simulink model "FinalRobot"  (R2021b)
settings: Solver=ode23t  StartTime=0.0  StopTime=120  MaxStep=3e-3  RelTol=1e-3
undefined symbols (not defined in the file): Amor1, Amor2, Amor3, Amor4, Amor5, B_Verin1, B_Verin2, B_Verin3, B_Verin4, B_Verin5, H_Verin1, H_Verin2, H_Verin3, H_Verin4, H_Verin5, k, K, Middle_Sensing, Sensing_1, Sensing_2, Wall_1, Wall_10, Wall_11, Wall_2, Wall_3, Wall_4, Wall_5, Wall_6, Wall_7, Wall_8, Wall_9, X, Y, Z
libraries: sm_lib x237, nesl_utility x60
(part 3 of 8)

== system FinalRobot/Snake/Verin2 ==
  Tor32 : Inport
  Torq31 : Inport  Port=2
  Camera : sm_lib/Body Elements/Spherical Solid  GraphicAmbientColor=[0.15 0.15 0.15 1.0]  BasedOnType=Density  CenterOfMass=[0 0 0]  CenterOfMassUnits=m  GraphicDiffuseColor=[0.9411765 0.9411765 0.9411765]  Density=10  DensityUnits=kg/m^3  DoExposeReferenceFrame=on  GraphicEmissiveColor=[0.0 0.0 0.0 1.0]  ExportEntireGeometry=off  SerializedExposedGeometries=<ExposedGeometries/>  SerializedFrames=<Frames/>  MarkerShape=Sphere  MarkerSize=10  GraphicType=FromGeometry  InertiaType=CalculateFromGeometry  Mass=1  MassUnits=kg  MomentsOfInertia=[1 1 1]  MomentsOfInertiaUnits=kg*m^2  GraphicOpacity=0  ProductsOfInertia=[0 0 0]  ProductsOfInertiaUnits=kg*m^2  GraphicShininess=75  GraphicSpecularColor=[0.5 0.5 0.5 1.0]  SphereRadius=0.1  SphereRadiusUnits=cm  GraphicVisPropType=SimpleVisualProperties
  Revolute Joint1 : sm_lib/Joints/Revolute Joint  JointMode=Normal  SenseConstraintForce=off  SenseConstraintForceX=off  SenseConstraintForceY=off  SenseConstraintForceZ=off  SenseConstraintTorque=off  SenseConstraintTorqueX=off  SenseConstraintTorqueY=off  SenseConstraintTorqueZ=off  SenseTotalForce=off  SenseTotalForceX=off  SenseTotalForceY=off  SenseTotalForceZ=off  SenseTotalTorque=off  SenseTotalTorqueX=off  SenseTotalTorqueY=off  SenseTotalTorqueZ=off  CompositeWrenchDir=FollowerOnBase  CompositeWrenchFrame=BaseFrame  EquilibriumPosition=0  EquilibriumPositionUnits=deg  SpringStiffness=Stiffness_Spine  SpringStiffnessUnits=N*m/deg  DampingCoefficient=Damping_Spine  DampingCoefficientUnits=N*m/(deg/s)  TorqueActuationMode=NoTorque  MotionActuationMode=ComputedMotion  SensePosition=off  SenseVelocity=off  SenseAcceleration=off  SenseTorqueForce=off  SenseLowerLimitTorqueForce=off  SenseUpperLimitTorqueForce=off  LowerLimitSpecify=off  LowerLimitBound=-90  LowerLimitBoundUnits=deg  LowerLimitStiffness=1e4  LowerLimitStiffnessUnits=N*m/deg  LowerLimitDamping=10  LowerLimitDampingUnits=N*m/(deg/s)  LowerLimitTransitionRegionWidth=0.1  LowerLimitTransitionRegionWidthUnits=deg  UpperLimitSpecify=off  UpperLimitBound=90  UpperLimitBoundUnits=deg  UpperLimitStiffness=1e4  UpperLimitStiffnessUnits=N*m/deg  UpperLimitDamping=10  UpperLimitDampingUnits=N*m/(deg/s)  UpperLimitTransitionRegionWidth=0.1  UpperLimitTransitionRegionWidthUnits=deg  PositionTargetSpecify=off  PositionTargetPriority=High  PositionTargetValue=0  PositionTargetValueUnits=deg  VelocityTargetSpecify=off  VelocityTargetPriority=High  VelocityTargetValue=0  VelocityTargetValueUnits=deg/s
  Rigid Transform4 : sm_lib/Frames and Transforms/Rigid Transform  TranslationMethod=Cartesian  TranslationStandardOffset=-10  TranslationLengthUnit=m  TranslationStandardAxis=+Z  TranslationCartesianOffset=[0 -0.1 0.1]  TranslationROffset=0  TranslationROffsetUnits=m  TranslationZOffset=0  TranslationZOffsetUnits=m  TranslationThetaOffset=0  TranslationThetaOffsetUnits=deg  RotationMethod=StandardAxis  RotationAngleUnits=deg  RotationStandardAxis=+Z  RotationAngle=-10  RotationArbitraryAxis=[0 0 1]  FollAlignAxisA=+X  BaseAlignAxisA=+Y  FollAlignAxisB=+Y  BaseAlignAxisB=+Z  RotationSequenceAxes=FollowerAxes  RotationSequence=XYX  RotationSequenceAngles=[-45 45 0]  RotationSequenceAnglesUnits=deg  RotationMatrix=[1 0 0; 0 1 0; 0 0 1]
  Subsystem1 : Subsystem
      mask Display: image('C:\Users\MINGO Monique\Pictures\MatLab images\MatLab_img3.PNG'); % Use "Edit Image" on toolstrip to change.
  Subsystem3 : Subsystem
      settings: PortSchema="{\"entries\":[{\"content\":{\"sides\":[{\"content\":{\"connectorIds\":[\"LConn1\"]},\"type\":\"ConnectorPlacement.EquallySpacedRectSide\",\"uuid\":\"fb7ca892-623b-4289-934f-aee105276814\"},{\"content\":{\"connectorIds\":[\"RConn1\"],\"side\":\"RIGHT\"},\"type\":\"ConnectorPlacement.EquallySpacedRectSide\",\"uuid\":\"0daf8b48-229f-46bb-9482-184447c743c5\"},{\"content\":{\"connectorIds\":[\"In1\",\"In2\",\"Out1\",\"Out2\"],\"side\":\"TOP\"},\"type\":\"ConnectorPlacement.EquallySpacedRectSide\",\"uuid\":\"c258a386-6c23-4ebb-b6ca-e534711f920f\"},{\"content\":{\"connectorIds\":[\"RConn2\",\"RConn3\",\"RConn4\",\"RConn5\"],\"side\":\"BOTTOM\"},\"type\":\"ConnectorPlacement.EquallySpacedRectSide\",\"uuid\":\"3e83ec0e-900d-4924-8cc6-19cde9453293\"}]},\"type\":\"ConnectorPlacement.EquallySpacedConnector\",\"uuid\":\"dfcdae3d-d414-45a1-b62e-1dc7d14d079d\"}],\"packageUris\":[\"http://schema.mathworks.com/mf0/Connector/R2020b\"],\"version\":\"1.0\"}"
      mask Display: image('$imagefile'); % Use "Edit Image" on toolstrip to change.
  Subsystem5 : Subsystem
      mask Display: image('C:\Users\MINGO Monique\Pictures\MatLab images\MatLab_img2.PNG'); % Use "Edit Image" on toolstrip to change.
  Conn1 : PMIOPort  Side=Left
  Conn7 : PMIOPort  Port=2  Side=Right
  Conn3 : PMIOPort  Port=3  Side=Right
  Amor : PMIOPort  Port=4  Side=Right
  Conn4 : PMIOPort  Port=5  Side=Right
  Conn2 : PMIOPort  Port=6  Side=Right
  Ref2 : PMIOPort  Port=7  Side=Right
  Ref3 : PMIOPort  Port=8  Side=Right
  azm3 : Outport
  wz3 : Outport  Port=2
  wires:
  Torq31/1 -> Subsystem3/2(input1)
  Tor32/1 -> Subsystem3/1(input0)
  Subsystem3/1(azm3) -> azm3/1
  Subsystem3/2(wz3) -> wz3/1
  connections:
  Subsystem3/RConn4 -- Conn2/RConn1
  Subsystem3/RConn3 -- Conn4/RConn1
  Subsystem3/RConn2 -- Amor/RConn1
  Conn7/RConn1 -- Subsystem1/LConn1 -- Subsystem3/RConn1
  Subsystem3/LConn1 -- Conn1/RConn1
  Conn3/RConn1 -- Rigid Transform4/LConn1 -- Subsystem5/RConn1
  Ref3/RConn1 -- Subsystem1/RConn1 -- Revolute Joint1/RConn1
  Revolute Joint1/LConn1 -- Subsystem5/LConn1
  Ref2/RConn1 -- Subsystem3/RConn5
  Camera/RConn1 -- Rigid Transform4/RConn1

== system FinalRobot/Snake/Verin3 ==
  Tor42 : Inport
  Torq41 : Inport  Port=2
  Revolute Joint1 : sm_lib/Joints/Revolute Joint  JointMode=Normal  SenseConstraintForce=off  SenseConstraintForceX=off  SenseConstraintForceY=off  SenseConstraintForceZ=off  SenseConstraintTorque=off  SenseConstraintTorqueX=off  SenseConstraintTorqueY=off  SenseConstraintTorqueZ=off  SenseTotalForce=off  SenseTotalForceX=off  SenseTotalForceY=off  SenseTotalForceZ=off  SenseTotalTorque=off  SenseTotalTorqueX=off  SenseTotalTorqueY=off  SenseTotalTorqueZ=off  CompositeWrenchDir=FollowerOnBase  CompositeWrenchFrame=BaseFrame  EquilibriumPosition=0  EquilibriumPositionUnits=deg  SpringStiffness=Stiffness_Spine  SpringStiffnessUnits=N*m/deg  DampingCoefficient=Damping_Spine  DampingCoefficientUnits=N*m/(deg/s)  TorqueActuationMode=NoTorque  MotionActuationMode=ComputedMotion  SensePosition=off  SenseVelocity=off  SenseAcceleration=off  SenseTorqueForce=off  SenseLowerLimitTorqueForce=off  SenseUpperLimitTorqueForce=off  LowerLimitSpecify=off  LowerLimitBound=-90  LowerLimitBoundUnits=deg  LowerLimitStiffness=1e4  LowerLimitStiffnessUnits=N*m/deg  LowerLimitDamping=10  LowerLimitDampingUnits=N*m/(deg/s)  LowerLimitTransitionRegionWidth=0.1  LowerLimitTransitionRegionWidthUnits=deg  UpperLimitSpecify=off  UpperLimitBound=90  UpperLimitBoundUnits=deg  UpperLimitStiffness=1e4  UpperLimitStiffnessUnits=N*m/deg  UpperLimitDamping=10  UpperLimitDampingUnits=N*m/(deg/s)  UpperLimitTransitionRegionWidth=0.1  UpperLimitTransitionRegionWidthUnits=deg  PositionTargetSpecify=off  PositionTargetPriority=High  PositionTargetValue=0  PositionTargetValueUnits=deg  VelocityTargetSpecify=off  VelocityTargetPriority=High  VelocityTargetValue=0  VelocityTargetValueUnits=deg/s
  Subsystem1 : Subsystem
      mask Display: image('C:\Users\MINGO Monique\Pictures\MatLab images\MatLab_img3.PNG'); % Use "Edit Image" on toolstrip to change.
  Subsystem3 : Subsystem
      settings: PortSchema="{\"entries\":[{\"content\":{\"sides\":[{\"content\":{\"connectorIds\":[\"LConn1\"]},\"type\":\"ConnectorPlacement.EquallySpacedRectSide\",\"uuid\":\"fb7ca892-623b-4289-934f-aee105276814\"},{\"content\":{\"connectorIds\":[\"RConn1\"],\"side\":\"RIGHT\"},\"type\":\"ConnectorPlacement.EquallySpacedRectSide\",\"uuid\":\"0daf8b48-229f-46bb-9482-184447c743c5\"},{\"content\":{\"connectorIds\":[\"In1\",\"In2\",\"Out1\",\"Out2\"],\"side\":\"TOP\"},\"type\":\"ConnectorPlacement.EquallySpacedRectSide\",\"uuid\":\"c258a386-6c23-4ebb-b6ca-e534711f920f\"},{\"content\":{\"connectorIds\":[\"RConn2\",\"RConn3\",\"RConn4\",\"RConn5\"],\"side\":\"BOTTOM\"},\"type\":\"ConnectorPlacement.EquallySpacedRectSide\",\"uuid\":\"3e83ec0e-900d-4924-8cc6-19cde9453293\"}]},\"type\":\"ConnectorPlacement.EquallySpacedConnector\",\"uuid\":\"dfcdae3d-d414-45a1-b62e-1dc7d14d079d\"}],\"packageUris\":[\"http://schema.mathworks.com/mf0/Connector/R2020b\"],\"version\":\"1.0\"}"
      mask Display: image('$imagefile'); % Use "Edit Image" on toolstrip to change.
  Subsystem5 : Subsystem
      mask Display: image('C:\Users\MINGO Monique\Pictures\MatLab images\MatLab_img2.PNG'); % Use "Edit Image" on toolstrip to change.
  Conn1 : PMIOPort  Side=Left
  Conn3 : PMIOPort  Port=2  Side=Right
  Amor : PMIOPort  Port=3  Side=Right
  Conn4 : PMIOPort  Port=4  Side=Right
  Conn2 : PMIOPort  Port=5  Side=Right
  Ref3 : PMIOPort  Port=6  Side=Right
  Ref4 : PMIOPort  Port=7  Side=Right
  azm4 : Outport
  wz4 : Outport  Port=2
  wires:
  Tor42/1 -> Subsystem3/1(input0)
  Torq41/1 -> Subsystem3/2(input1)
  Subsystem3/1(azm4) -> azm4/1
  Subsystem3/2(wz4) -> wz4/1
  connections:
  Subsystem3/LConn1 -- Conn1/RConn1
  Subsystem3/RConn2 -- Amor/RConn1
  Subsystem3/RConn3 -- Conn4/RConn1
  Subsystem3/RConn4 -- Conn2/RConn1
  Ref4/RConn1 -- Subsystem1/RConn1 -- Revolute Joint1/RConn1
  Revolute Joint1/LConn1 -- Subsystem5/LConn1
  Subsystem1/LConn1 -- Subsystem3/RConn1
  Ref3/RConn1 -- Subsystem3/RConn5
  Conn3/RConn1 -- Subsystem5/RConn1

== system FinalRobot/Snake/Verin4 ==
  Tor52 : Inport
  Torq51 : Inport  Port=2
  Subsystem1 : Subsystem
      settings: PortSchema="{\"entries\":[{\"content\":{\"sides\":[{\"content\":{\"connectorIds\":[\"LConn1\"]},\"type\":\"ConnectorPlacement.EquallySpacedRectSide\",\"uuid\":\"fb7ca892-623b-4289-934f-aee105276814\"},{\"content\":{\"connectorIds\":[\"RConn1\"],\"side\":\"RIGHT\"},\"type\":\"ConnectorPlacement.EquallySpacedRectSide\",\"uuid\":\"0daf8b48-229f-46bb-9482-184447c743c5\"},{\"content\":{\"connectorIds\":[\"In1\",\"In2\",\"Out1\",\"Out2\"],\"side\":\"TOP\"},\"type\":\"ConnectorPlacement.EquallySpacedRectSide\",\"uuid\":\"c258a386-6c23-4ebb-b6ca-e534711f920f\"},{\"content\":{\"connectorIds\":[\"RConn2\",\"RConn3\",\"RConn4\",\"RConn5\"],\"side\":\"BOTTOM\"},\"type\":\"ConnectorPlacement.EquallySpacedRectSide\",\"uuid\":\"3e83ec0e-900d-4924-8cc6-19cde9453293\"}]},\"type\":\"ConnectorPlacement.EquallySpacedConnector\",\"uuid\":\"dfcdae3d-d414-45a1-b62e-1dc7d14d079d\"}],\"packageUris\":[\"http://schema.mathworks.com/mf0/Connector/R2020b\"],\"version\":\"1.0\"}"
      mask Display: image('$imagefile'); % Use "Edit Image" on toolstrip to change.
  Conn1 : PMIOPort  Side=Left
  Amor : PMIOPort  Port=2  Side=Right
  Conn4 : PMIOPort  Port=3  Side=Right
  Conn2 : PMIOPort  Port=4  Side=Right
  Ref4 : PMIOPort  Port=5  Side=Right
  azm5 : Outport
  wz5 : Outport  Port=2
  wires:
  Torq51/1 -> Subsystem1/2(input1)
  Tor52/1 -> Subsystem1/1(input0)
  Subsystem1/1(azm5) -> azm5/1
  Subsystem1/2(wz5) -> wz5/1
  connections:
  Subsystem1/RConn4 -- Conn2/RConn1
  Subsystem1/RConn3 -- Conn4/RConn1
  Subsystem1/RConn2 -- Amor/RConn1
  Subsystem1/LConn1 -- Conn1/RConn1
  Ref4/RConn1 -- Subsystem1/RConn5

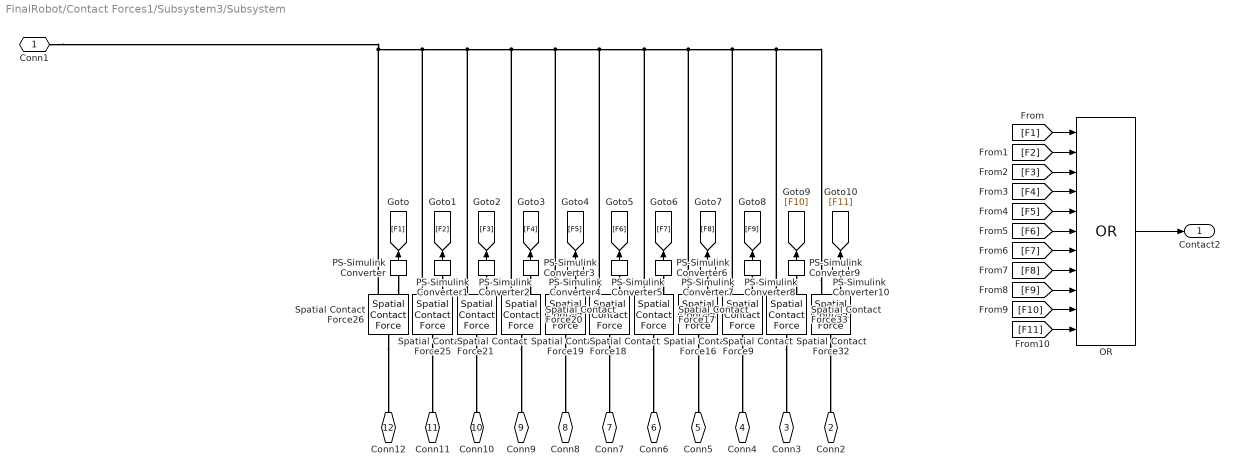
== system FinalRobot/Contact Forces1/Subsystem3/Subsystem ==
  OR : Logic  Operator=OR  Inputs=11  IconShape=distinctive  AllPortsSameDT=off  OutDataTypeStr=boolean
  PS-Simulink Converter{,1..10} (11 alike) : nesl_utility/PS-Simulink Converter  PhysicalDomain=network_engine_domain  SubClassName=ps_output  LeftPortType=input  RightPortType=output  PseudoPeriodic=off  Frequencies=[]  Unit=inherit  AffineConversion=off
      settings: SourceProductBaseCode=PW,SS
  Spatial Contact Force{9,16..21,25..26,32..33} (11 alike) : sm_lib/Forces and Torques/Spatial Contact Force  CoefficientOfDynamicFriction=0.3  CoefficientOfStaticFriction=0.5  SenseContactBaseRotation=off  SenseContactBaseTranslation=off  NormalDamping=1e3  NormalDampingUnits=N/(m/s)  SenseContactFollowerRotation=off  SenseContactFollowerTranslation=off  SenseContactSignal=off  NormalStiffness=1e6  NormalStiffnessUnits=N/m  FrictionalCriticalVelocity=1e-3  FrictionalCriticalVelocityUnits=m/s  ZeroCrossDetectContactStartAndEnd=off  FrictionType=SmoothStickSlip  SenseFrictionalForceMagnitude=off  SenseNormalForceMagnitude=on  NormalForceType=SmoothSpringDamper  SenseNormalVelocity=off  SenseSeparationDistance=off  SenseTangentialVelocity=off  SenseTangentialVelocityMagnitude=off  NormalTransitionRegionWidth=1e-4  NormalTransitionRegionWidthUnits=m
  Conn1 : PMIOPort  Side=Left
  Conn2 : PMIOPort  Port=2  Side=Right
  Conn3 : PMIOPort  Port=3  Side=Right
  Conn4 : PMIOPort  Port=4  Side=Right
  Conn5 : PMIOPort  Port=5  Side=Right
  Conn6 : PMIOPort  Port=6  Side=Right
  Conn7 : PMIOPort  Port=7  Side=Right
  Conn8 : PMIOPort  Port=8  Side=Right
  Conn9 : PMIOPort  Port=9  Side=Right
  Conn10 : PMIOPort  Port=10  Side=Right
  Conn11 : PMIOPort  Port=11  Side=Right
  Conn12 : PMIOPort  Port=12  Side=Right
  Contact2 : Outport
  wires:
  PS-Simulink Converter8/1 -> [F9]
  PS-Simulink Converter9/1 -> [F10]
  [F11] -> OR/11
  [F7] -> OR/7
  [F6] -> OR/6
  PS-Simulink Converter1/1 -> [F2]
  OR/1 -> Contact2/1
  [F2] -> OR/2
  PS-Simulink Converter4/1 -> [F5]
  [F4] -> OR/4
  PS-Simulink Converter7/1 -> [F8]
  [F10] -> OR/10
  [F3] -> OR/3
  [F1] -> OR/1
  PS-Simulink Converter2/1 -> [F3]
  PS-Simulink Converter3/1 -> [F4]
  [F8] -> OR/8
  PS-Simulink Converter/1 -> [F1]
  PS-Simulink Converter10/1 -> [F11]
  [F9] -> OR/9
  PS-Simulink Converter6/1 -> [F7]
  PS-Simulink Converter5/1 -> [F6]
  [F5] -> OR/5
  connections:
  Spatial Contact Force33/LConn1 -- Conn3/RConn1
  PS-Simulink Converter6/LConn1 -- Spatial Contact Force17/RConn2
  PS-Simulink Converter4/LConn1 -- Spatial Contact Force19/RConn2
  Spatial Contact Force9/RConn2 -- PS-Simulink Converter8/LConn1
  PS-Simulink Converter9/LConn1 -- Spatial Contact Force33/RConn2
  Spatial Contact Force18/LConn1 -- Conn7/RConn1
  PS-Simulink Converter1/LConn1 -- Spatial Contact Force25/RConn2
  Spatial Contact Force32/RConn1 -- Conn1/RConn1 -- Spatial Contact Force26/RConn1 -- Spatial Contact Force25/RConn1 -- Spatial Contact Force21/RConn1 -- Spatial Contact Force20/RConn1 -- Spatial Contact Force19/RConn1 -- Spatial Contact Force18/RConn1 -- Spatial Contact Force17/RConn1 -- Spatial Contact Force16/RConn1 -- Spatial Contact Force9/RConn1 -- Spatial Contact Force33/RConn1
  PS-Simulink Converter7/LConn1 -- Spatial Contact Force16/RConn2
  Spatial Contact Force16/LConn1 -- Conn5/RConn1
  PS-Simulink Converter5/LConn1 -- Spatial Contact Force18/RConn2
  Spatial Contact Force20/LConn1 -- Conn9/RConn1
  PS-Simulink Converter2/LConn1 -- Spatial Contact Force21/RConn2
  PS-Simulink Converter/LConn1 -- Spatial Contact Force26/RConn2
  Spatial Contact Force21/LConn1 -- Conn10/RConn1
  Spatial Contact Force17/LConn1 -- Conn6/RConn1
  Spatial Contact Force19/LConn1 -- Conn8/RConn1
  PS-Simulink Converter10/LConn1 -- Spatial Contact Force32/RConn2
  PS-Simulink Converter3/LConn1 -- Spatial Contact Force20/RConn2
  Spatial Contact Force25/LConn1 -- Conn11/RConn1
  Spatial Contact Force26/LConn1 -- Conn12/RConn1
  Spatial Contact Force32/LConn1 -- Conn2/RConn1
  Spatial Contact Force9/LConn1 -- Conn4/RConn1

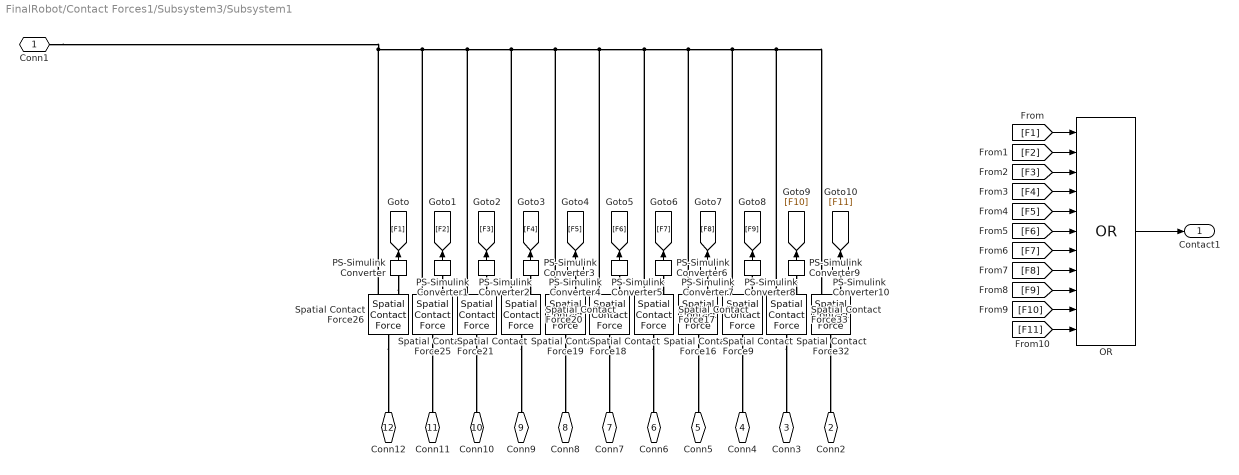
== system FinalRobot/Contact Forces1/Subsystem3/Subsystem1 ==
  OR : Logic  Operator=OR  Inputs=11  IconShape=distinctive  AllPortsSameDT=off  OutDataTypeStr=boolean
  PS-Simulink Converter{,1..10} (11 alike) : nesl_utility/PS-Simulink Converter  PhysicalDomain=network_engine_domain  SubClassName=ps_output  LeftPortType=input  RightPortType=output  PseudoPeriodic=off  Frequencies=[]  Unit=inherit  AffineConversion=off
      settings: SourceProductBaseCode=PW,SS
  Spatial Contact Force{9,16..21,25..26,32..33} (11 alike) : sm_lib/Forces and Torques/Spatial Contact Force  CoefficientOfDynamicFriction=0.3  CoefficientOfStaticFriction=0.5  SenseContactBaseRotation=off  SenseContactBaseTranslation=off  NormalDamping=1e3  NormalDampingUnits=N/(m/s)  SenseContactFollowerRotation=off  SenseContactFollowerTranslation=off  SenseContactSignal=off  NormalStiffness=1e6  NormalStiffnessUnits=N/m  FrictionalCriticalVelocity=1e-3  FrictionalCriticalVelocityUnits=m/s  ZeroCrossDetectContactStartAndEnd=off  FrictionType=SmoothStickSlip  SenseFrictionalForceMagnitude=off  SenseNormalForceMagnitude=on  NormalForceType=SmoothSpringDamper  SenseNormalVelocity=off  SenseSeparationDistance=off  SenseTangentialVelocity=off  SenseTangentialVelocityMagnitude=off  NormalTransitionRegionWidth=1e-4  NormalTransitionRegionWidthUnits=m
  Conn1 : PMIOPort  Side=Left
  Conn2 : PMIOPort  Port=2  Side=Right
  Conn3 : PMIOPort  Port=3  Side=Right
  Conn4 : PMIOPort  Port=4  Side=Right
  Conn5 : PMIOPort  Port=5  Side=Right
  Conn6 : PMIOPort  Port=6  Side=Right
  Conn7 : PMIOPort  Port=7  Side=Right
  Conn8 : PMIOPort  Port=8  Side=Right
  Conn9 : PMIOPort  Port=9  Side=Right
  Conn10 : PMIOPort  Port=10  Side=Right
  Conn11 : PMIOPort  Port=11  Side=Right
  Conn12 : PMIOPort  Port=12  Side=Right
  Contact1 : Outport
  wires:
  [F5] -> OR/5
  PS-Simulink Converter5/1 -> [F6]
  PS-Simulink Converter6/1 -> [F7]
  [F9] -> OR/9
  PS-Simulink Converter10/1 -> [F11]
  PS-Simulink Converter/1 -> [F1]
  [F8] -> OR/8
  PS-Simulink Converter3/1 -> [F4]
  PS-Simulink Converter2/1 -> [F3]
  [F1] -> OR/1
  [F3] -> OR/3
  [F10] -> OR/10
  PS-Simulink Converter7/1 -> [F8]
  [F4] -> OR/4
  PS-Simulink Converter4/1 -> [F5]
  [F2] -> OR/2
  OR/1 -> Contact1/1
  PS-Simulink Converter1/1 -> [F2]
  [F6] -> OR/6
  [F7] -> OR/7
  [F11] -> OR/11
  PS-Simulink Converter9/1 -> [F10]
  PS-Simulink Converter8/1 -> [F9]
  connections:
  Spatial Contact Force9/LConn1 -- Conn4/RConn1
  Spatial Contact Force32/LConn1 -- Conn2/RConn1
  Spatial Contact Force26/LConn1 -- Conn12/RConn1
  Spatial Contact Force25/LConn1 -- Conn11/RConn1
  PS-Simulink Converter3/LConn1 -- Spatial Contact Force20/RConn2
  PS-Simulink Converter10/LConn1 -- Spatial Contact Force32/RConn2
  Spatial Contact Force19/LConn1 -- Conn8/RConn1
  Spatial Contact Force17/LConn1 -- Conn6/RConn1
  Spatial Contact Force21/LConn1 -- Conn10/RConn1
  PS-Simulink Converter/LConn1 -- Spatial Contact Force26/RConn2
  PS-Simulink Converter2/LConn1 -- Spatial Contact Force21/RConn2
  Spatial Contact Force20/LConn1 -- Conn9/RConn1
  PS-Simulink Converter5/LConn1 -- Spatial Contact Force18/RConn2
  Spatial Contact Force16/LConn1 -- Conn5/RConn1
  PS-Simulink Converter7/LConn1 -- Spatial Contact Force16/RConn2
  Conn1/RConn1 -- Spatial Contact Force32/RConn1 -- Spatial Contact Force33/RConn1 -- Spatial Contact Force9/RConn1 -- Spatial Contact Force16/RConn1 -- Spatial Contact Force17/RConn1 -- Spatial Contact Force18/RConn1 -- Spatial Contact Force19/RConn1 -- Spatial Contact Force20/RConn1 -- Spatial Contact Force21/RConn1 -- Spatial Contact Force25/RConn1 -- Spatial Contact Force26/RConn1
  PS-Simulink Converter1/LConn1 -- Spatial Contact Force25/RConn2
  Spatial Contact Force18/LConn1 -- Conn7/RConn1
  PS-Simulink Converter9/LConn1 -- Spatial Contact Force33/RConn2
  Spatial Contact Force9/RConn2 -- PS-Simulink Converter8/LConn1
  PS-Simulink Converter4/LConn1 -- Spatial Contact Force19/RConn2
  PS-Simulink Converter6/LConn1 -- Spatial Contact Force17/RConn2
  Spatial Contact Force33/LConn1 -- Conn3/RConn1

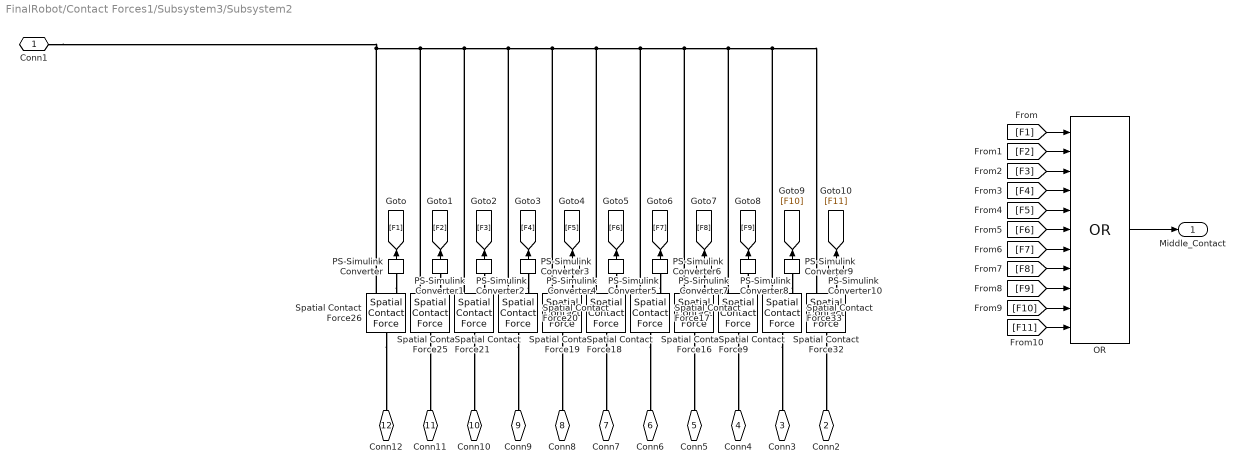
== system FinalRobot/Contact Forces1/Subsystem3/Subsystem2 ==
  OR : Logic  Operator=OR  Inputs=11  IconShape=distinctive  AllPortsSameDT=off  OutDataTypeStr=boolean
  PS-Simulink Converter{,1..10} (11 alike) : nesl_utility/PS-Simulink Converter  PhysicalDomain=network_engine_domain  SubClassName=ps_output  LeftPortType=input  RightPortType=output  PseudoPeriodic=off  Frequencies=[]  Unit=inherit  AffineConversion=off
      settings: SourceProductBaseCode=PW,SS
  Spatial Contact Force{9,16..21,25..26,32..33} (11 alike) : sm_lib/Forces and Torques/Spatial Contact Force  CoefficientOfDynamicFriction=0.3  CoefficientOfStaticFriction=0.5  SenseContactBaseRotation=off  SenseContactBaseTranslation=off  NormalDamping=1e3  NormalDampingUnits=N/(m/s)  SenseContactFollowerRotation=off  SenseContactFollowerTranslation=off  SenseContactSignal=off  NormalStiffness=1e6  NormalStiffnessUnits=N/m  FrictionalCriticalVelocity=1e-3  FrictionalCriticalVelocityUnits=m/s  ZeroCrossDetectContactStartAndEnd=off  FrictionType=SmoothStickSlip  SenseFrictionalForceMagnitude=off  SenseNormalForceMagnitude=on  NormalForceType=SmoothSpringDamper  SenseNormalVelocity=off  SenseSeparationDistance=off  SenseTangentialVelocity=off  SenseTangentialVelocityMagnitude=off  NormalTransitionRegionWidth=1e-4  NormalTransitionRegionWidthUnits=m
  Conn1 : PMIOPort  Side=Left
  Conn2 : PMIOPort  Port=2  Side=Right
  Conn3 : PMIOPort  Port=3  Side=Right
  Conn4 : PMIOPort  Port=4  Side=Right
  Conn5 : PMIOPort  Port=5  Side=Right
  Conn6 : PMIOPort  Port=6  Side=Right
  Conn7 : PMIOPort  Port=7  Side=Right
  Conn8 : PMIOPort  Port=8  Side=Right
  Conn9 : PMIOPort  Port=9  Side=Right
  Conn10 : PMIOPort  Port=10  Side=Right
  Conn11 : PMIOPort  Port=11  Side=Right
  Conn12 : PMIOPort  Port=12  Side=Right
  Middle_Contact : Outport
  wires:
  PS-Simulink Converter8/1 -> [F9]
  PS-Simulink Converter9/1 -> [F10]
  [F11] -> OR/11
  [F7] -> OR/7
  [F6] -> OR/6
  PS-Simulink Converter1/1 -> [F2]
  OR/1 -> Middle_Contact/1
  [F2] -> OR/2
  PS-Simulink Converter4/1 -> [F5]
  [F4] -> OR/4
  PS-Simulink Converter7/1 -> [F8]
  [F10] -> OR/10
  [F3] -> OR/3
  [F1] -> OR/1
  PS-Simulink Converter2/1 -> [F3]
  PS-Simulink Converter3/1 -> [F4]
  [F8] -> OR/8
  PS-Simulink Converter/1 -> [F1]
  PS-Simulink Converter10/1 -> [F11]
  [F9] -> OR/9
  PS-Simulink Converter6/1 -> [F7]
  PS-Simulink Converter5/1 -> [F6]
  [F5] -> OR/5
  connections:
  Spatial Contact Force33/LConn1 -- Conn3/RConn1
  PS-Simulink Converter6/LConn1 -- Spatial Contact Force17/RConn2
  PS-Simulink Converter4/LConn1 -- Spatial Contact Force19/RConn2
  Spatial Contact Force9/RConn2 -- PS-Simulink Converter8/LConn1
  PS-Simulink Converter9/LConn1 -- Spatial Contact Force33/RConn2
  Spatial Contact Force18/LConn1 -- Conn7/RConn1
  PS-Simulink Converter1/LConn1 -- Spatial Contact Force25/RConn2
  Spatial Contact Force26/RConn1 -- Spatial Contact Force25/RConn1 -- Spatial Contact Force21/RConn1 -- Spatial Contact Force20/RConn1 -- Spatial Contact Force19/RConn1 -- Spatial Contact Force18/RConn1 -- Spatial Contact Force17/RConn1 -- Spatial Contact Force16/RConn1 -- Spatial Contact Force9/RConn1 -- Spatial Contact Force33/RConn1 -- Spatial Contact Force32/RConn1 -- Conn1/RConn1
  PS-Simulink Converter7/LConn1 -- Spatial Contact Force16/RConn2
  Spatial Contact Force16/LConn1 -- Conn5/RConn1
  PS-Simulink Converter5/LConn1 -- Spatial Contact Force18/RConn2
  Spatial Contact Force20/LConn1 -- Conn9/RConn1
  PS-Simulink Converter2/LConn1 -- Spatial Contact Force21/RConn2
  PS-Simulink Converter/LConn1 -- Spatial Contact Force26/RConn2
  Spatial Contact Force21/LConn1 -- Conn10/RConn1
  Spatial Contact Force17/LConn1 -- Conn6/RConn1
  Spatial Contact Force19/LConn1 -- Conn8/RConn1
  PS-Simulink Converter10/LConn1 -- Spatial Contact Force32/RConn2
  PS-Simulink Converter3/LConn1 -- Spatial Contact Force20/RConn2
  Spatial Contact Force25/LConn1 -- Conn11/RConn1
  Spatial Contact Force26/LConn1 -- Conn12/RConn1
  Spatial Contact Force32/LConn1 -- Conn2/RConn1
  Spatial Contact Force9/LConn1 -- Conn4/RConn1

== system FinalRobot/Snake/Verin/Subsystem2 ==
  input0 : Inport
  Cylindrical Solid3 : sm_lib/Body Elements/Cylindrical Solid  GraphicAmbientColor=[0.15 0.15 0.15 1.0]  BasedOnType=Density  CenterOfMass=[0 0 0]  CenterOfMassUnits=m  GraphicDiffuseColor=[0.5 0.5 0.5]  CylinderLength=2  CylinderLengthUnits=cm  CylinderRadius=1.5  CylinderRadiusUnits=cm  Density=1000  DensityUnits=kg/m^3  DoExposeReferenceFrame=off  GraphicEmissiveColor=[0.0 0.0 0.0 1.0]  ExportEntireGeometry=off  SerializedFrames=<Frames><Frame><Id>Frame1</Id><Value><Name>F1</Name><Origin><Source>GeometricFeature</Source><FeatureName>bottom curve</FeatureName></Origin><PrimaryAxis><DefinedDirection>+Z</DefinedDirection><Source>ReferenceFrame</Source><SourceDirection>+Y</SourceDirection><FeatureName></FeatureName></PrimaryAxis><SecondaryAxis><DefinedDirection>+X</DefinedDirection><Source>ReferenceFrame</Source><SourceDirection>+Z</SourceDirection><FeatureName></FeatureName></SecondaryAxis></Value></Frame><Frame><Id>Frame2</Id><Value><Name>F2</Name><Origin><Source>GeometricFeature</Source><FeatureName>top curve</FeatureName></Origin><PrimaryAxis><DefinedDirection>+Z</DefinedDirection><Source>ReferenceFrame</Source><SourceDirection>+Y</SourceDirection><FeatureName></FeatureName></PrimaryAxis><SecondaryAxis><DefinedDirection>+X</DefinedDirection><Source>ReferenceFrame</Source><SourceDirection>+Z</SourceDirection><FeatureName></FeatureName></SecondaryAxis></Value></Frame></Frames>  MarkerShape=Sphere  MarkerSize=10  GraphicType=FromGeometry  InertiaType=CalculateFromGeometry  Mass=1  MassUnits=kg  MomentsOfInertia=[1 1 1]  MomentsOfInertiaUnits=kg*m^2  GraphicOpacity=1.0  ProductsOfInertia=[0 0 0]  ProductsOfInertiaUnits=kg*m^2  GraphicShininess=75  GraphicSpecularColor=[0.5 0.5 0.5 1.0]  GraphicVisPropType=SimpleVisualProperties
  Cylindrical Solid4 : sm_lib/Body Elements/Cylindrical Solid  GraphicAmbientColor=[0.15 0.15 0.15 1.0]  BasedOnType=Density  CenterOfMass=[0 0 0]  CenterOfMassUnits=m  GraphicDiffuseColor=[0.5 0.5 0.5]  CylinderLength=3  CylinderLengthUnits=cm  CylinderRadius=1.5  CylinderRadiusUnits=cm  Density=1000  DensityUnits=kg/m^3  DoExposeReferenceFrame=off  GraphicEmissiveColor=[0.0 0.0 0.0 1.0]  ExportEntireGeometry=off  SerializedFrames=<Frames><Frame><Id>Frame1</Id><Value><Name>F1</Name><Origin><Source>GeometricFeature</Source><FeatureName>bottom curve</FeatureName></Origin><PrimaryAxis><DefinedDirection>+Z</DefinedDirection><Source>ReferenceFrame</Source><SourceDirection>+Y</SourceDirection><FeatureName></FeatureName></PrimaryAxis><SecondaryAxis><DefinedDirection>+X</DefinedDirection><Source>ReferenceFrame</Source><SourceDirection>+Z</SourceDirection><FeatureName></FeatureName></SecondaryAxis></Value></Frame><Frame><Id>Frame2</Id><Value><Name>F2</Name><Origin><Source>GeometricFeature</Source><FeatureName>top curve</FeatureName></Origin><PrimaryAxis><DefinedDirection>+Z</DefinedDirection><Source>ReferenceFrame</Source><SourceDirection>+Y</SourceDirection><FeatureName></FeatureName></PrimaryAxis><SecondaryAxis><DefinedDirection>+X</DefinedDirection><Source>ReferenceFrame</Source><SourceDirection>+Z</SourceDirection><FeatureName></FeatureName></SecondaryAxis></Value></Frame></Frames>  MarkerShape=Sphere  MarkerSize=10  GraphicType=FromGeometry  InertiaType=CalculateFromGeometry  Mass=1  MassUnits=kg  MomentsOfInertia=[1 1 1]  MomentsOfInertiaUnits=kg*m^2  GraphicOpacity=1.0  ProductsOfInertia=[0 0 0]  ProductsOfInertiaUnits=kg*m^2  GraphicShininess=75  GraphicSpecularColor=[0.5 0.5 0.5 1.0]  GraphicVisPropType=SimpleVisualProperties
  Cylindrical Solid5 : sm_lib/Body Elements/Cylindrical Solid  GraphicAmbientColor=[0.15 0.15 0.15 1.0]  BasedOnType=Density  CenterOfMass=[0 0 0]  CenterOfMassUnits=m  GraphicDiffuseColor=[0.5 0.5 0.5]  CylinderLength=5.2  CylinderLengthUnits=cm  CylinderRadius=2  CylinderRadiusUnits=cm  Density=1000  DensityUnits=kg/m^3  DoExposeReferenceFrame=off  GraphicEmissiveColor=[0.0 0.0 0.0 1.0]  ExportEntireGeometry=off  SerializedFrames=<Frames><Frame><Id>Frame1</Id><Value><Name>F1</Name><Origin><Source>ReferenceFrame</Source><FeatureName></FeatureName></Origin><PrimaryAxis><DefinedDirection>+Z</DefinedDirection><Source>ReferenceFrame</Source><SourceDirection>+Z</SourceDirection><FeatureName></FeatureName></PrimaryAxis><SecondaryAxis><DefinedDirection>+X</DefinedDirection><Source>ReferenceFrame</Source><SourceDirection>-X</SourceDirection><FeatureName></FeatureName></SecondaryAxis></Value></Frame></Frames>  MarkerShape=Sphere  MarkerSize=10  GraphicType=FromGeometry  InertiaType=CalculateFromGeometry  Mass=1  MassUnits=kg  MomentsOfInertia=[1 1 1]  MomentsOfInertiaUnits=kg*m^2  GraphicOpacity=1.0  ProductsOfInertia=[0 0 0]  ProductsOfInertiaUnits=kg*m^2  GraphicShininess=75  GraphicSpecularColor=[0.5 0.5 0.5 1.0]  GraphicVisPropType=SimpleVisualProperties
  Extruded Solid : sm_lib/Body Elements/Extruded Solid  GraphicAmbientColor=[0.15 0.15 0.15 1.0]  BasedOnType=Density  CenterOfMass=[0 0 0]  CenterOfMassUnits=m  GraphicDiffuseColor=[1.0 1.0 1.0]  ExportConvexHullGeometry=off  ExtrusionCrossSection=elev_joint_1  ExtrusionCrossSectionUnits=cm  Density=1000  DensityUnits=kg/m^3  DoExposeReferenceFrame=on  GraphicEmissiveColor=[0.0 0.0 0.0 1.0]  ExportEntireGeometry=off  ExtrusionLength=1.1  ExtrusionLengthUnits=cm  ExtrusionType=General  SerializedFrames=<Frames/>  MarkerShape=Sphere  MarkerSize=10  GraphicType=FromGeometry  InertiaType=CalculateFromGeometry  Mass=1  MassUnits=kg  MomentsOfInertia=[1 1 1]  MomentsOfInertiaUnits=kg*m^2  PolygonNumSides=3  GraphicOpacity=1.0  PolygonOuterRadius=1  PolygonOuterRadiusUnits=m  ProductsOfInertia=[0 0 0]  ProductsOfInertiaUnits=kg*m^2  GraphicShininess=75  GraphicSpecularColor=[0.5 0.5 0.5 1.0]  GraphicVisPropType=SimpleVisualProperties
  Extruded Solid1 : sm_lib/Body Elements/Extruded Solid  GraphicAmbientColor=[0.15 0.15 0.15 1.0]  BasedOnType=Density  CenterOfMass=[0 0 0]  CenterOfMassUnits=m  GraphicDiffuseColor=[1.0 1.0 1.0]  ExportConvexHullGeometry=off  ExtrusionCrossSection=elev_joint_1  ExtrusionCrossSectionUnits=cm  Density=1000  DensityUnits=kg/m^3  DoExposeReferenceFrame=on  GraphicEmissiveColor=[0.0 0.0 0.0 1.0]  ExportEntireGeometry=off  ExtrusionLength=1.1  ExtrusionLengthUnits=cm  ExtrusionType=General  SerializedFrames=<Frames/>  MarkerShape=Sphere  MarkerSize=10  GraphicType=FromGeometry  InertiaType=CalculateFromGeometry  Mass=1  MassUnits=kg  MomentsOfInertia=[1 1 1]  MomentsOfInertiaUnits=kg*m^2  PolygonNumSides=3  GraphicOpacity=1.0  PolygonOuterRadius=1  PolygonOuterRadiusUnits=m  ProductsOfInertia=[0 0 0]  ProductsOfInertiaUnits=kg*m^2  GraphicShininess=75  GraphicSpecularColor=[0.5 0.5 0.5 1.0]  GraphicVisPropType=SimpleVisualProperties
  Extruded Solid2 : sm_lib/Body Elements/Extruded Solid  GraphicAmbientColor=[0.15 0.15 0.15 1.0]  BasedOnType=Density  CenterOfMass=[0 0 0]  CenterOfMassUnits=m  GraphicDiffuseColor=[1.0 1.0 1.0]  ExportConvexHullGeometry=off  ExtrusionCrossSection=elev_joint_2  ExtrusionCrossSectionUnits=cm  Density=1000  DensityUnits=kg/m^3  DoExposeReferenceFrame=on  GraphicEmissiveColor=[0.0 0.0 0.0 1.0]  ExportEntireGeometry=off  ExtrusionLength=3  ExtrusionLengthUnits=cm  ExtrusionType=General  SerializedFrames=<Frames><Frame><Id>Frame1</Id><Value><Name>F</Name><Origin><Source>ReferenceFrame</Source><FeatureName></FeatureName></Origin><PrimaryAxis><DefinedDirection>+Z</DefinedDirection><Source>ReferenceFrame</Source><SourceDirection>+Z</SourceDirection><FeatureName></FeatureName></PrimaryAxis><SecondaryAxis><DefinedDirection>+X</DefinedDirection><Source>ReferenceFrame</Source><SourceDirection>-X</SourceDirection><FeatureName></FeatureName></SecondaryAxis></Value></Frame></Frames>  MarkerShape=Sphere  MarkerSize=10  GraphicType=FromGeometry  InertiaType=CalculateFromGeometry  Mass=1  MassUnits=kg  MomentsOfInertia=[1 1 1]  MomentsOfInertiaUnits=kg*m^2  PolygonNumSides=3  GraphicOpacity=1.0  PolygonOuterRadius=1  PolygonOuterRadiusUnits=m  ProductsOfInertia=[0 0 0]  ProductsOfInertiaUnits=kg*m^2  GraphicShininess=75  GraphicSpecularColor=[0.5 0.5 0.5 1.0]  GraphicVisPropType=SimpleVisualProperties
  Revolute Joint1 : sm_lib/Joints/Revolute Joint  JointMode=Normal  SenseConstraintForce=off  SenseConstraintForceX=off  SenseConstraintForceY=off  SenseConstraintForceZ=off  SenseConstraintTorque=off  SenseConstraintTorqueX=off  SenseConstraintTorqueY=off  SenseConstraintTorqueZ=off  SenseTotalForce=off  SenseTotalForceX=off  SenseTotalForceY=off  SenseTotalForceZ=off  SenseTotalTorque=off  SenseTotalTorqueX=off  SenseTotalTorqueY=off  SenseTotalTorqueZ=off  CompositeWrenchDir=FollowerOnBase  CompositeWrenchFrame=BaseFrame  EquilibriumPosition=0  EquilibriumPositionUnits=deg  SpringStiffness=1.337  SpringStiffnessUnits=N*m/rad  DampingCoefficient=1.337  DampingCoefficientUnits=N*m/(rad/s)  TorqueActuationMode=ComputedTorque  MotionActuationMode=InputMotion  SensePosition=off  SenseVelocity=off  SenseAcceleration=off  SenseTorqueForce=off  SenseLowerLimitTorqueForce=off  SenseUpperLimitTorqueForce=off  LowerLimitSpecify=on  LowerLimitBound=-90  LowerLimitBoundUnits=deg  LowerLimitStiffness=1e4  LowerLimitStiffnessUnits=N*m/deg  LowerLimitDamping=10  LowerLimitDampingUnits=N*m/(deg/s)  LowerLimitTransitionRegionWidth=0.1  LowerLimitTransitionRegionWidthUnits=deg  UpperLimitSpecify=on  UpperLimitBound=90  UpperLimitBoundUnits=deg  UpperLimitStiffness=1e4  UpperLimitStiffnessUnits=N*m/deg  UpperLimitDamping=10  UpperLimitDampingUnits=N*m/(deg/s)  UpperLimitTransitionRegionWidth=0.1  UpperLimitTransitionRegionWidthUnits=deg  PositionTargetSpecify=off  PositionTargetPriority=High  PositionTargetValue=0  PositionTargetValueUnits=deg  VelocityTargetSpecify=off  VelocityTargetPriority=High  VelocityTargetValue=0  VelocityTargetValueUnits=deg/s
  Rigid Transform1 : sm_lib/Frames and Transforms/Rigid Transform  TranslationMethod=StandardAxis  TranslationStandardOffset=2  TranslationLengthUnit=cm  TranslationStandardAxis=-X  TranslationCartesianOffset=[0 0 0]  TranslationROffset=0  TranslationROffsetUnits=m  TranslationZOffset=0  TranslationZOffsetUnits=m  TranslationThetaOffset=0  TranslationThetaOffsetUnits=deg  RotationMethod=None  RotationAngleUnits=deg  RotationStandardAxis=+Z  RotationAngle=0.0  RotationArbitraryAxis=[0 0 1]  FollAlignAxisA=+X  BaseAlignAxisA=+Y  FollAlignAxisB=+Y  BaseAlignAxisB=+Z  RotationSequenceAxes=FollowerAxes  RotationSequence=XYX  RotationSequenceAngles=[0 0 0]  RotationSequenceAnglesUnits=deg  RotationMatrix=[1 0 0; 0 1 0; 0 0 1]
  Rigid Transform2 : sm_lib/Frames and Transforms/Rigid Transform  TranslationMethod=StandardAxis  TranslationStandardOffset=1.5  TranslationLengthUnit=cm  TranslationStandardAxis=+Z  TranslationCartesianOffset=[0 0 0]  TranslationROffset=0  TranslationROffsetUnits=m  TranslationZOffset=0  TranslationZOffsetUnits=m  TranslationThetaOffset=0  TranslationThetaOffsetUnits=deg  RotationMethod=None  RotationAngleUnits=deg  RotationStandardAxis=+Z  RotationAngle=0.0  RotationArbitraryAxis=[0 0 1]  FollAlignAxisA=+X  BaseAlignAxisA=+Y  FollAlignAxisB=+Y  BaseAlignAxisB=+Z  RotationSequenceAxes=FollowerAxes  RotationSequence=XYX  RotationSequenceAngles=[0 0 0]  RotationSequenceAnglesUnits=deg  RotationMatrix=[1 0 0; 0 1 0; 0 0 1]
  Rigid Transform3 : sm_lib/Frames and Transforms/Rigid Transform  TranslationMethod=StandardAxis  TranslationStandardOffset=1.5  TranslationLengthUnit=cm  TranslationStandardAxis=-Z  TranslationCartesianOffset=[0 0 0]  TranslationROffset=0  TranslationROffsetUnits=m  TranslationZOffset=0  TranslationZOffsetUnits=m  TranslationThetaOffset=0  TranslationThetaOffsetUnits=deg  RotationMethod=None  RotationAngleUnits=deg  RotationStandardAxis=+Z  RotationAngle=0.0  RotationArbitraryAxis=[0 0 1]  FollAlignAxisA=+X  BaseAlignAxisA=+Y  FollAlignAxisB=+Y  BaseAlignAxisB=+Z  RotationSequenceAxes=FollowerAxes  RotationSequence=XYX  RotationSequenceAngles=[0 0 0]  RotationSequenceAnglesUnits=deg  RotationMatrix=[1 0 0; 0 1 0; 0 0 1]
  Rigid Transform5 : sm_lib/Frames and Transforms/Rigid Transform  TranslationMethod=StandardAxis  TranslationStandardOffset=0.55  TranslationLengthUnit=cm  TranslationStandardAxis=-Z  TranslationCartesianOffset=[0 0 0]  TranslationROffset=0  TranslationROffsetUnits=m  TranslationZOffset=0  TranslationZOffsetUnits=m  TranslationThetaOffset=0  TranslationThetaOffsetUnits=deg  RotationMethod=None  RotationAngleUnits=deg  RotationStandardAxis=+Z  RotationAngle=0.0  RotationArbitraryAxis=[0 0 1]  FollAlignAxisA=+X  BaseAlignAxisA=+Y  FollAlignAxisB=+Y  BaseAlignAxisB=+Z  RotationSequenceAxes=FollowerAxes  RotationSequence=XYX  RotationSequenceAngles=[0 0 0]  RotationSequenceAnglesUnits=deg  RotationMatrix=[1 0 0; 0 1 0; 0 0 1]
  Rigid Transform6 : sm_lib/Frames and Transforms/Rigid Transform  TranslationMethod=StandardAxis  TranslationStandardOffset=0.55  TranslationLengthUnit=cm  TranslationStandardAxis=+Z  TranslationCartesianOffset=[0 0 0]  TranslationROffset=0  TranslationROffsetUnits=m  TranslationZOffset=0  TranslationZOffsetUnits=m  TranslationThetaOffset=0  TranslationThetaOffsetUnits=deg  RotationMethod=None  RotationAngleUnits=deg  RotationStandardAxis=+Z  RotationAngle=0.0  RotationArbitraryAxis=[0 0 1]  FollAlignAxisA=+X  BaseAlignAxisA=+Y  FollAlignAxisB=+Y  BaseAlignAxisB=+Z  RotationSequenceAxes=FollowerAxes  RotationSequence=XYX  RotationSequenceAngles=[0 0 0]  RotationSequenceAnglesUnits=deg  RotationMatrix=[1 0 0; 0 1 0; 0 0 1]
  Simulink-PS Converter2 : nesl_utility/Simulink-PS Converter  PhysicalDomain=network_engine_domain  SubClassName=ps_input  LeftPortType=input  RightPortType=output  PseudoPeriodic=off  Frequencies=[]  NoiseDistribution=none  NoiseParameters=[]  Unit=1  AffineConversion=off  FilteringAndDerivatives=filter  SimscapeFilterOrder=2  InputFilterTimeConstant=0.001  UdotUserProvided=0
      settings: SourceProductBaseCode=PW,SS
  Conn2 : PMIOPort  Side=Left
  Conn1 : PMIOPort  Port=2  Side=Right
  Ref1 : PMIOPort  Port=3  Side=Right
  wires:
  input0/1 -> Simulink-PS Converter2/1
  connections:
  Extruded Solid/RConn1 -- Rigid Transform5/LConn1
  Extruded Solid1/RConn1 -- Rigid Transform6/LConn1
  Cylindrical Solid3/LConn1 -- Conn1/RConn1
  Rigid Transform1/RConn1 -- Cylindrical Solid3/RConn1
  Extruded Solid2/LConn1 -- Rigid Transform1/LConn1 -- Revolute Joint1/LConn1
  Cylindrical Solid4/LConn1 -- Ref1/RConn1 -- Revolute Joint1/RConn1 -- Cylindrical Solid5/LConn1
  Conn2/RConn1 -- Cylindrical Solid4/RConn1
  Simulink-PS Converter2/RConn1 -- Revolute Joint1/LConn2
  Rigid Transform5/RConn1 -- Rigid Transform2/RConn1
  Rigid Transform2/LConn1 -- Extruded Solid2/RConn1 -- Rigid Transform3/LConn1
  Rigid Transform3/RConn1 -- Rigid Transform6/RConn1
